simulink subsystem "thermal_subsystem_model_stage_3"  (R2023a)
settings: Solver=VariableStepAuto  StartTime=0.0  StopTime=10.0  RelTol=1e-3
values from neighbouring files (symbols this model uses):
  air_cp = 1004    [thermal_harness_parameters.m]
  air_HC_min = 10    [thermal_harness_parameters.m]
  air_HC_nom = 100    [thermal_harness_parameters.m]
  air_rho = 1.2    [thermal_harness_parameters.m]
  air_vel_nom = 1    [thermal_harness_parameters.m]
  coolant_initial_pressure = 0.111325    [thermal_model_parameters.m]    (also in thermal_plant_h2f175_parameters.m)
  coolant_initial_temperature = 293.15    [thermal_model_parameters.m]    (also in thermal_plant_h2f175_parameters.m)
  coolant_tube_D = 0.05    [thermal_model_parameters.m]    (also in thermal_plant_h2f175_parameters.m)
  radiator_area_air = radiator_n_fins * radiator_fin_height * radiator_fin_width    (= 0.1026)    [thermal_harness_parameters.m]
  radiator_area_fins = radiator_n_fins * (radiator_fin_height-radiator_fin_thickness) * radiator_width * 2    (= 2.543625)    [thermal_harness_parameters.m]
  radiator_area_primary = 2 * radiator_tube_length * radiator_width * (radiator_fin_rows)     - 2 * radiator_fin_thickness * radiator_width * radiator_n_fins     + 2 * radiator_fin_height * radiator_width * radiator_fin_rows     + 2 * radiator_tube_height * radiator_n_tubes * radiator_tube_length    [thermal_harness_parameters.m]
  radiator_n_tubes = 20    [thermal_harness_parameters.m]
  radiator_tube_height = 0.0015    [thermal_harness_parameters.m]
  radiator_tube_length = 0.45    [thermal_harness_parameters.m]
  radiator_width = 0.025    [thermal_harness_parameters.m]
  tcp_time_constant = 2    [thermal_model_parameters.m]    (also in thermal_plant_h2f175_parameters.m)
  tcv_orifice_diameter = 0.045    [thermal_model_parameters.m]    (also in thermal_plant_h2f175_parameters.m)
  tcv_time_constant = .2    (= 0.2)    [thermal_model_parameters.m]    (also in thermal_plant_h2f175_parameters.m)
libraries: fl_lib x50, nesl_utility x40, SimscapeFluids_lib x8
(part 2 of 2)

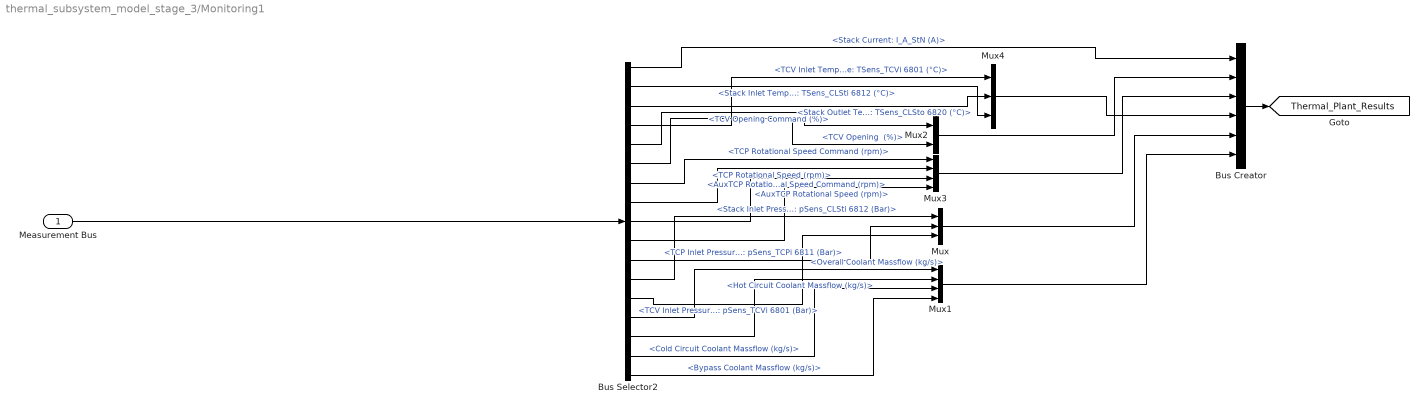
== system thermal_subsystem_model_stage_3/Monitoring1 ==
  Measurement Bus : Inport
  Bus Creator : BusCreator  Inputs=6
  Bus Selector2 : BusSelector  OutputSignals="Stack Current: I_A_StN (A),Stack Inlet Temperature: TSens_CLSti 6812 (°C),Stack Outlet Temperature: TSens_CLSto 6820 (°C),TCV Inlet Temperature: TSens_TCVi 6801 (°C),TCV Opening Command (%),TCV Opening  (%),TCP Rotational Speed Command (rpm),TCP Rotational Speed (rpm),AuxTCP Rotational Speed Command (rpm),AuxTCP Rotational Speed (rpm),TCP Inlet Pressure: pSens_TCPi 6811 (Bar),Stack Inlet Pressure: pSens_CLSti 6812 (Bar),TCV Inlet Pressure: pSens_TCVi 6801 (Bar),Overall Coolant Massflow (kg/s),Hot Circuit Coolant Massflow (kg/s),Cold Circuit Coolant Massflow (kg/s),Bypass Coolant Massflow (kg/s)"
  Mux : Mux  Inputs=3
  Mux1 : Mux
  Mux2 : Mux  Inputs=2
  Mux3 : Mux
  Mux4 : Mux  Inputs=3
  tag scope: Thermal_Plant_Results=global
  wires:
  Bus Creator/1 -> [Thermal_Plant_Results]
  Bus Selector2/4 -> Mux4/1  "<TCV Inlet Temperature: TSens_TCVi 6801 (°C)>"
  Bus Selector2/1 -> Bus Creator/1  "<Stack Current: I_A_StN (A)>"
  Bus Selector2/12 -> Mux/1  "<Stack Inlet Pressure: pSens_CLSti 6812 (Bar)>"
  Bus Selector2/16 -> Mux1/3  "<Cold Circuit Coolant Massflow (kg/s)>"
  Bus Selector2/5 -> Mux2/1  "<TCV Opening Command (%)>"
  Bus Selector2/8 -> Mux3/2  "<TCP Rotational Speed (rpm)>"
  Bus Selector2/17 -> Mux1/4  "<Bypass Coolant Massflow (kg/s)>"
  Mux1/1 -> Bus Creator/6
  Bus Selector2/14 -> Mux1/1  "<Overall Coolant Massflow (kg/s)>"
  Bus Selector2/13 -> Mux/3  "<TCV Inlet Pressure: pSens_TCVi 6801 (Bar)>"
  Bus Selector2/15 -> Mux1/2  "<Hot Circuit Coolant Massflow (kg/s)>"
  Mux/1 -> Bus Creator/5
  Bus Selector2/6 -> Mux2/2  "<TCV Opening  (%)>"
  Bus Selector2/2 -> Mux4/3  "<Stack Inlet Temperature: TSens_CLSti 6812 (°C)>"
  Bus Selector2/9 -> Mux3/3  "<AuxTCP Rotational Speed Command (rpm)>"
  Measurement Bus/1 -> Bus Selector2/1
  Mux2/1 -> Bus Creator/2
  Bus Selector2/3 -> Mux4/2  "<Stack Outlet Temperature: TSens_CLSto 6820 (°C)>"
  Bus Selector2/7 -> Mux3/1  "<TCP Rotational Speed Command (rpm)>"
  Mux3/1 -> Bus Creator/3
  Bus Selector2/11 -> Mux/2  "<TCP Inlet Pressure: pSens_TCPi 6811 (Bar)>"
  Mux4/1 -> Bus Creator/4
  Bus Selector2/10 -> Mux3/4  "<AuxTCP Rotational Speed (rpm)>"

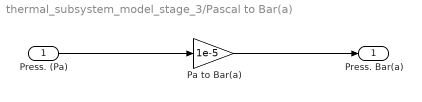
== system thermal_subsystem_model_stage_3/Pascal to Bar(a) ==
  Press. (Pa) : Inport
  Pa to Bar(a) : Gain  Gain=1e-5
  Press. Bar(a) : Outport
  wires:
  Press. (Pa)/1 -> Pa to Bar(a)/1
  Pa to Bar(a)/1 -> Press. Bar(a)/1

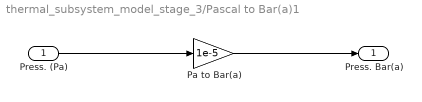
== system thermal_subsystem_model_stage_3/Pascal to Bar(a)1 ==
  Press. (Pa) : Inport
  Pa to Bar(a) : Gain  Gain=1e-5
  Press. Bar(a) : Outport
  wires:
  Press. (Pa)/1 -> Pa to Bar(a)/1
  Pa to Bar(a)/1 -> Press. Bar(a)/1

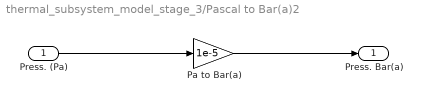
== system thermal_subsystem_model_stage_3/Pascal to Bar(a)2 ==
  Press. (Pa) : Inport
  Pa to Bar(a) : Gain  Gain=1e-5
  Press. Bar(a) : Outport
  wires:
  Press. (Pa)/1 -> Pa to Bar(a)/1
  Pa to Bar(a)/1 -> Press. Bar(a)/1

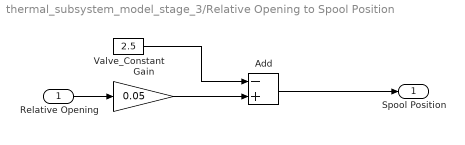
== system thermal_subsystem_model_stage_3/Relative Opening to Spool Position ==
  Relative Opening : Inport
  Add : Sum  Inputs=-+
  Gain : Gain  Gain=0.05
  Valve_Constant : Constant  Value=2.5
  Spool Position : Outport
  wires:
  Add/1 -> Spool Position/1
  Valve_Constant/1 -> Add/1
  Relative Opening/1 -> Gain/1
  Gain/1 -> Add/2
